simulink model "LANDER_mutibodymodel0x2810x29"  (R2024b)
settings: Solver=VariableStepAuto  StartTime=0.0  StopTime=20  RelTol=1e-3
undefined symbols (not defined in the file): X, Y, Z
libraries: sm_lib x58, nesl_utility x10
(part 1 of 4)
settings Model: Creator=dipayan  LastModifiedBy=tirth
settings RTWCC: GPUComputeCapability=3.5

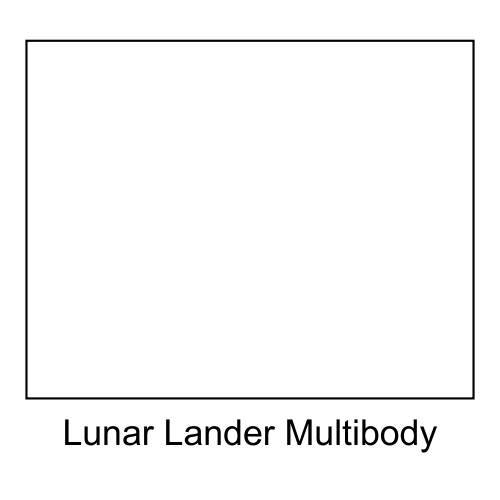
[thumbnail: Simulink's stored preview of the top-level diagram]
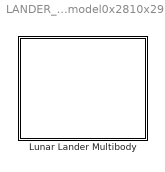
== system LANDER_mutibodymodel0x2810x29 ==
  Lunar Lander Multibody : Subsystem

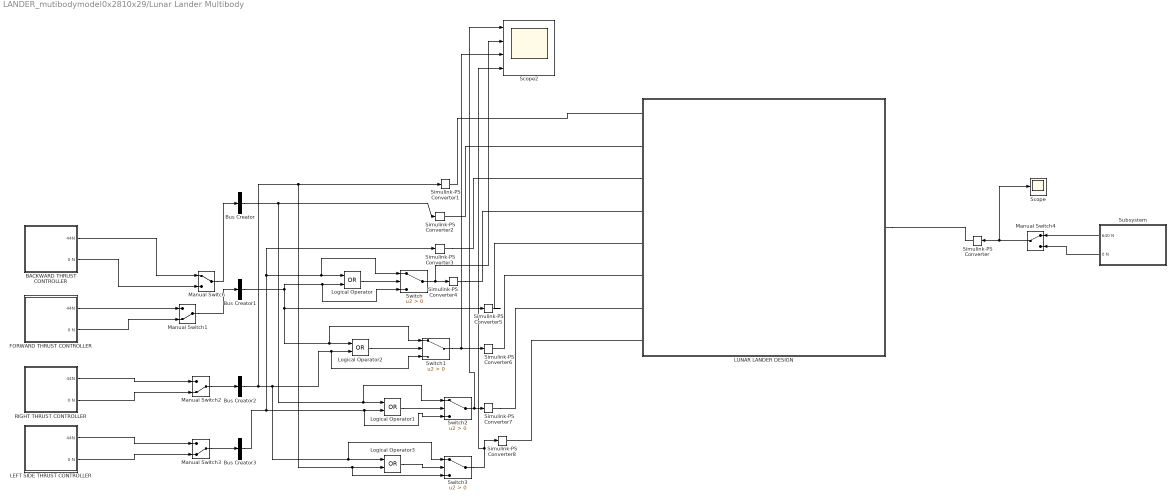
== system LANDER_mutibodymodel0x2810x29/Lunar Lander Multibody ==
  " BACKWARD THRUST CONTROLLER" : Subsystem
  " FORWARD THRUST CONTROLLER" : Subsystem
  Bus Creator{,1..3} (4 alike) : BusCreator  Inputs=1
  LEFT SIDE THRUST CONTROLLER : Subsystem
  LUNAR LANDER DESIGN : Subsystem
  Logical Operator{,1..3} (4 alike) : Logic  Operator=OR  AllPortsSameDT=off  OutDataTypeStr=boolean
  Manual Switch : ManualSwitch
  Manual Switch1 : ManualSwitch  CurrentSetting=0
  Manual Switch2 : ManualSwitch  CurrentSetting=0
  Manual Switch3 : ManualSwitch  CurrentSetting=0
  Manual Switch4 : ManualSwitch
  RIGHT THRUST CONTROLLER : Subsystem
  Scope : Scope
  Scope2 : Scope  NumInputPorts=4
  Simulink-PS Converter{,1..8} (9 alike) : nesl_utility/Simulink-PS Converter  PhysicalDomain=network_engine_domain  SubClassName=ps_input  LeftPortType=input  RightPortType=output  PseudoPeriodic=off  Frequencies=[]  NoiseDistribution=none  NoiseParameters=[]  Unit=1  AffineConversion=off  FilteringAndDerivatives=provide  SimscapeFilterOrder=1  InputFilterTimeConstant=0.001  UdotUserProvided=0
  Subsystem : Subsystem
  Switch{,1..3} (4 alike) : Switch  Criteria=u2 > Threshold  SaturateOnIntegerOverflow=off  InputSameDT=off
  wires:
  Switch1/1 -> Simulink-PS Converter6/1, Scope2/3
  Switch2/1 -> Simulink-PS Converter7/1, Scope2/1
  Switch3/1 -> Scope2/4, Simulink-PS Converter8/1
  Manual Switch/1 -> Bus Creator/1
  " BACKWARD THRUST CONTROLLER"/1(44N) -> Manual Switch/1
  " BACKWARD THRUST CONTROLLER"/2(0 N) -> Manual Switch/2
  " FORWARD THRUST CONTROLLER"/1(44N) -> Manual Switch1/1
  " FORWARD THRUST CONTROLLER"/2(0 N) -> Manual Switch1/2
  Manual Switch1/1 -> Bus Creator1/1
  Manual Switch2/1 -> Bus Creator2/1
  RIGHT THRUST CONTROLLER/1(44N) -> Manual Switch2/1
  RIGHT THRUST CONTROLLER/2(0 N) -> Manual Switch2/2
  Manual Switch3/1 -> Bus Creator3/1
  LEFT SIDE THRUST CONTROLLER/1(44N) -> Manual Switch3/1
  LEFT SIDE THRUST CONTROLLER/2(0 N) -> Manual Switch3/2
  Switch/1 -> Scope2/2, Simulink-PS Converter4/1
  Bus Creator2/1 -> Switch3/1, Logical Operator3/1, Logical Operator2/2, Switch1/3, Simulink-PS Converter1/1, Switch3/3, Logical Operator3/2
  Bus Creator1/1 -> Logical Operator2/1, Switch1/1, Simulink-PS Converter5/1, Logical Operator/2, Switch/3
  Logical Operator2/1 -> Switch1/2
  Logical Operator/1 -> Switch/2
  Logical Operator1/1 -> Switch2/2
  Bus Creator3/1 -> Logical Operator1/2, Switch2/3, Simulink-PS Converter3/1, Logical Operator/1, Switch/1
  Bus Creator/1 -> Logical Operator1/1, Switch2/1, Simulink-PS Converter2/1
  Logical Operator3/1 -> Switch3/2
  Manual Switch4/1 -> Scope/1, Simulink-PS Converter/1
  Subsystem/1(640 N) -> Manual Switch4/1
  Subsystem/2(0 N) -> Manual Switch4/2
  connections:
  LUNAR LANDER DESIGN/RConn1 -- Simulink-PS Converter/RConn1
  Simulink-PS Converter1/RConn1 -- LUNAR LANDER DESIGN/LConn1
  LUNAR LANDER DESIGN/LConn2 -- Simulink-PS Converter2/RConn1
  Simulink-PS Converter3/RConn1 -- LUNAR LANDER DESIGN/LConn3
  Simulink-PS Converter4/RConn1 -- LUNAR LANDER DESIGN/LConn4
  Simulink-PS Converter7/RConn1 -- LUNAR LANDER DESIGN/LConn7
  LUNAR LANDER DESIGN/LConn8 -- Simulink-PS Converter8/RConn1
  Simulink-PS Converter5/RConn1 -- LUNAR LANDER DESIGN/LConn5
  LUNAR LANDER DESIGN/LConn6 -- Simulink-PS Converter6/RConn1

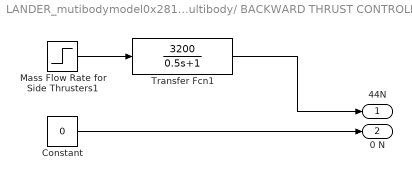
== system LANDER_mutibodymodel0x2810x29/Lunar Lander Multibody/ BACKWARD THRUST CONTROLLER ==
  Constant : Constant  Value=0
  Mass Flow Rate for Side Thrusters1 : Step  Time=0  After=0.01375  SampleTime=0
  Transfer Fcn1 : TransferFcn  Numerator=[3200]  Denominator=[0.5 1]
  44N : Outport
  0 N : Outport  Port=2
  wires:
  Mass Flow Rate for Side Thrusters1/1 -> Transfer Fcn1/1
  Transfer Fcn1/1 -> 44N/1
  Constant/1 -> 0 N/1

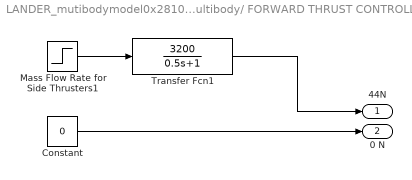
== system LANDER_mutibodymodel0x2810x29/Lunar Lander Multibody/ FORWARD THRUST CONTROLLER ==
  Constant : Constant  Value=0
  Mass Flow Rate for Side Thrusters1 : Step  Time=0  After=0.01375  SampleTime=0
  Transfer Fcn1 : TransferFcn  Numerator=[3200]  Denominator=[0.5 1]
  44N : Outport
  0 N : Outport  Port=2
  wires:
  Mass Flow Rate for Side Thrusters1/1 -> Transfer Fcn1/1
  Transfer Fcn1/1 -> 44N/1
  Constant/1 -> 0 N/1

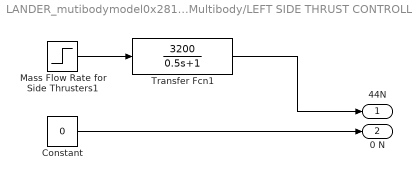
== system LANDER_mutibodymodel0x2810x29/Lunar Lander Multibody/LEFT SIDE THRUST CONTROLLER ==
  Constant : Constant  Value=0
  Mass Flow Rate for Side Thrusters1 : Step  Time=0  After=0.01375  SampleTime=0
  Transfer Fcn1 : TransferFcn  Numerator=[3200]  Denominator=[0.5 1]
  44N : Outport
  0 N : Outport  Port=2
  wires:
  Mass Flow Rate for Side Thrusters1/1 -> Transfer Fcn1/1
  Transfer Fcn1/1 -> 44N/1
  Constant/1 -> 0 N/1
